simulink model "clean_pendulum_math_model2"  (R2020b)
settings: Solver=FixedStepAuto  StartTime=0.0  StopTime=100.0  FixedStep=0.01  RelTol=1e-3
values from neighbouring files (symbols this model uses):
  f_c = 1.0942    [clean_pendulum_setup.m]
  f_p = 0.10436    [clean_pendulum_setup.m]
  g = 9.8101    [Wahadlo_setup.m]    (also in clean_pendulum_setup.m = 9.81)
  I = 1/12 * m_pw * l_c ^ 2      + 1/4 * m_pw * r_c ^ 2      + m_pw * l_c0 ^ 2      + 1/12 * m_ps * l_p ^ 2      + 1/4 * m_pw * r_p ^ 2      + m_ps * l_p0 ^ 2    (= 0.00542605689)    [clean_pendulum_setup.m]
  L = 0.2899    [clean_pendulum_setup.m]
  M = 0.503 + 0.045    (= 0.548)    [clean_pendulum_setup.m]
  m = m_c + m_p    (= 63.548)    [Wahadlo_setup.m]    (also in clean_pendulum_setup.m = 0.063)
settings Model: Creator=spika  LastModifiedBy=spika

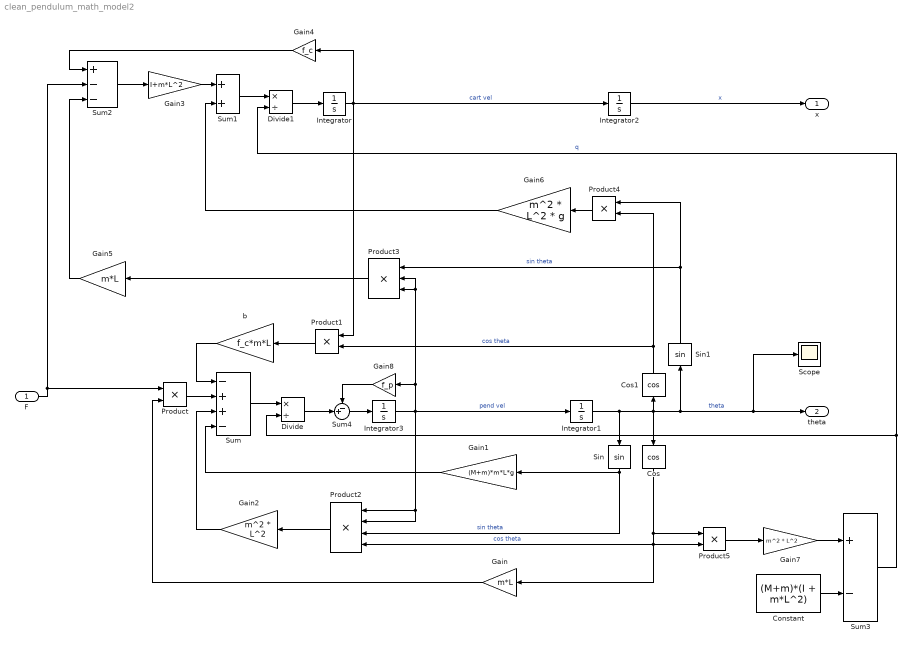
== system clean_pendulum_math_model2 ==
  F : Inport
  Constant : Constant  Value=(M+m)*(I + m*L^2)
  Cos : Trigonometry  Operator=cos
  Cos1 : Trigonometry  Operator=cos
  Divide : Product  Inputs=*/
  Divide1 : Product  Inputs=*/
  Gain : Gain  Gain=m*L
  Gain1 : Gain  Gain=(M+m)*m*L*g
  Gain2 : Gain  Gain=m^2 * L^2
  Gain3 : Gain  Gain=I+m*L^2
  Gain4 : Gain  Gain=f_c
  Gain5 : Gain  Gain=m*L
  Gain6 : Gain  Gain=m^2 * L^2 * g
  Gain7 : Gain  Gain=m^2 * L^2
  Gain8 : Gain  Gain=f_p
  Integrator : Integrator
  Integrator1 : Integrator  InitialCondition=0.1
  Integrator2 : Integrator
  Integrator3 : Integrator
  Product{,1,4..5} (4 alike) : Product
  Product2 : Product  Inputs=4
  Product3 : Product  Inputs=3
  Scope : Scope
  Sin : Trigonometry
  Sin1 : Trigonometry
  Sum : Sum  Inputs=-++-
  Sum1 : Sum
  Sum2 : Sum  Inputs=+--
  Sum3 : Sum  Inputs=+-
  Sum4 : Sum  Inputs=-+|
  b : Gain  Gain=f_c*m*L
  x : Outport
  theta : Outport  Port=2
  wires:
  Integrator/1 -> Gain4/1, Integrator2/1, Product1/1  "cart vel"
  Integrator3/1 -> Product3/2, Product3/3, Gain8/1, Integrator1/1, Product2/1, Product2/2  "pend vel"
  Integrator2/1 -> x/1  "x"
  Integrator1/1 -> Cos1/1, Scope/1, theta/1, Sin1/1, Cos/1, Sin/1  "theta"
  F/1 -> Sum2/2, Product/1
  Gain/1 -> Product/2
  Cos/1 -> Product5/1, Product5/2, Product2/4, Gain/1  "cos theta"
  Cos1/1 -> Product4/2, Product1/2  "cos theta"
  Product1/1 -> b/1
  b/1 -> Sum/1
  Sin/1 -> Product2/3, Gain1/1  "sin theta"
  Product/1 -> Sum/2
  Gain1/1 -> Sum/4
  Product2/1 -> Gain2/1
  Gain2/1 -> Sum/3
  Sum2/1 -> Gain3/1
  Gain4/1 -> Sum2/1
  Sin1/1 -> Product4/1, Product3/1  "sin theta"
  Product3/1 -> Gain5/1
  Gain5/1 -> Sum2/3
  Gain3/1 -> Sum1/1
  Product4/1 -> Gain6/1
  Gain6/1 -> Sum1/2
  Product5/1 -> Gain7/1
  Gain7/1 -> Sum3/1
  Constant/1 -> Sum3/2
  Sum/1 -> Divide/1
  Sum3/1 -> Divide1/2, Divide/2  "q"
  Divide1/1 -> Integrator/1
  Sum1/1 -> Divide1/1
  Divide/1 -> Sum4/2
  Sum4/1 -> Integrator3/1
  Gain8/1 -> Sum4/1
